simulink model "vec_ut"  (Simulink 8.1)
settings: Solver=FixedStepDiscrete  StartTime=0.0  StopTime=10  FixedStep=0.005  RelTol=1e-3
PostLoadFcn:
  | , if any(exist('dsrtsu_mdlpostloadfcn', 'file') == [2, 3, 6]), try dsrtsu_mdlpostloadfcn('Execute', bdroot); catch fprintf('Error in PostLoadFcn (dsrtsu_mdlpostloadfcn) for model "%s":\n %s\n', bdroot, lasterr); end, end,
libraries: siltestlib x4, idiada_lib x4, vec x1
settings Model: DSRTSU_INTERNAL_RTI_VER=450  DSRTSU_INTERNAL_RTI_TYPE=rti1401  RTICANMMDATA=struct('GeneralSetupData',struct('modelroot','D:\ELN150201_TAIWAN\trunk\AdasDragon\software\sw_development\arch\app\ifo','generalsettings',struct('filesettings',struct('destfolder',struct('Name','RTICANMM_FILES','Check',1),'buildfolder',struct('Name','.','Check',1),'AbsDestfolder',struct('Name','D:\ELN150201_TAIWAN\trunk\AdasDragon\software\sw_development\arch\app\ifo\RTICANMM_FILES'),'AbsBuildfolder',struct('Name','D:\ELN150201_TAIWAN\trunk\AdasDragon\software\sw_development\arch\app\ifo'))),'options',struct('addpaths',1,'rmpaths',1,'addtrcexclusion',logical(1),'cannavigator',struct('checkmonitoring',0),'show_usrtrc',0,'use_usrtrc',0),'advanced',struct('options',[1 1 1 1 1 1 1 1 1 1 1 1 1 1 1 1 1 1 1 1 1 1 1 1 1 1 1 1 1 1 1 1 1 1 1 1 1 1 1 1 1 1 1 1 1 1 1 1 1 1 1 1 1 1 1 1 1 1 1 1 1 1 1 1 1 1 1 1 1 1 1 1 1 1 1 1 1 1 1 1 1 1 1 1 1 1 1 1 1 1 1 1 1 1 1 1 1 1 1 1]),'MPSetup',{{}},'modelname','vec_ut','block','vec_ut'))  DSRTSU_INTERNAL_RTIFPGA=40  Creator=AT015411  LastModifiedBy=AT015555  BufferReuse=off
settings DataIOCC: SignalLoggingSaveFormat=Dataset
settings OptimizationCC: BlockReduction=off  OptimizeBlockIOStorage=off  BufferReuse=off  ExpressionFolding=off  ExpressionDepthLimit=128  LocalBlockOutputs=off
settings DebuggingCC: FcnCallInpInsideContextMsg=EnableAllAsError
settings HardwareCC: ProdIntDivRoundTo=Zero  ProdEndianess=BigEndian  ProdHWDeviceType=Generic->Custom  TargetIntDivRoundTo=Zero  TargetEndianess=BigEndian  TargetHWDeviceType=Generic->Custom
settings RTWCC: SystemTargetFile=rti1005.tlc  MakeCommand=make_rti  TemplateMakefile=rti1005.tmf  Description=dSPACE DS1005 Hardware Platform  ProcessScript=rti1005_make_rtw_hook
settings STFCustomTargetCC: CodeReplacementLibrary=ANSI_C  ParMdlRefBuildCompliant=on  GeneratePreprocessorConditionals=Disable all  MatFileLogging=on  SystemTargetFile=rti1005.tlc
settings GRTTargetCC: CompOptLevelCompliant=off  ConcurrentExecutionCompliant=off  ExtModeMexFile=noextcomm
settings CustomProperty: DataType=RTWOptions_EnumType_C__Program Files (x86)_dSPACE RCPHIL 2014-B_MATLAB_RTI_RTI1401_TLC_rti1005_1InitialSimState  Value=RUN
settings EnumStrPairs: String=RUN

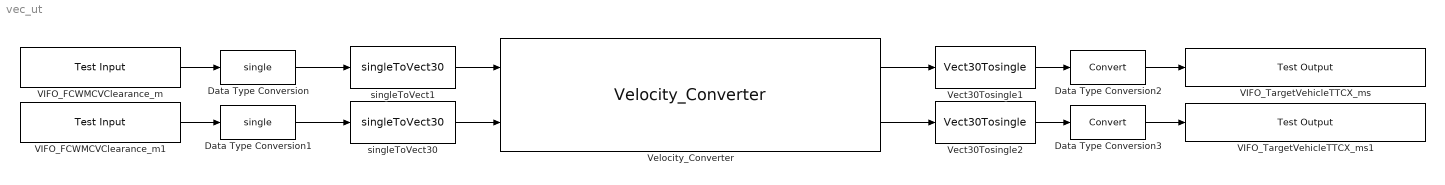
== system vec_ut ==
  Data Type Conversion : DataTypeConversion  OutDataTypeStr=single
  Data Type Conversion1 : DataTypeConversion  OutDataTypeStr=single
  Data Type Conversion2 : DataTypeConversion
  Data Type Conversion3 : DataTypeConversion
  VIFO_FCWMCVClearance_m : siltestlib/Test Input  varname=VPER_TargAbsSpeedVect30_mps  sampletime=0.005
  VIFO_FCWMCVClearance_m1 : siltestlib/Test Input  varname=VPER_TargAttitudeVect30_rad  sampletime=0.005
  VIFO_TargetVehicleTTCX_ms : siltestlib/Test Output  varname=VIFO_TargAbsSpeedXVect30_mps  sampletime=-1
  VIFO_TargetVehicleTTCX_ms1 : siltestlib/Test Output  varname=VIFO_TargAbsSpeedYVect30_mps  sampletime=-1
  Vect30Tosingle1 : idiada_lib/Vect30Tosingle
  Vect30Tosingle2 : idiada_lib/Vect30Tosingle
  Velocity_Converter : vec/Velocity_Converter
  singleToVect1 : idiada_lib/singleToVect30
  singleToVect30 : idiada_lib/singleToVect30
  wires:
  VIFO_FCWMCVClearance_m/1 -> Data Type Conversion/1
  Velocity_Converter/1 -> Vect30Tosingle1/1
  Data Type Conversion2/1 -> VIFO_TargetVehicleTTCX_ms/1
  Data Type Conversion/1 -> singleToVect1/1
  VIFO_FCWMCVClearance_m1/1 -> Data Type Conversion1/1
  Data Type Conversion1/1 -> singleToVect30/1
  Velocity_Converter/2 -> Vect30Tosingle2/1
  Data Type Conversion3/1 -> VIFO_TargetVehicleTTCX_ms1/1
  singleToVect30/1 -> Velocity_Converter/2
  singleToVect1/1 -> Velocity_Converter/1
  Vect30Tosingle1/1 -> Data Type Conversion2/1
  Vect30Tosingle2/1 -> Data Type Conversion3/1
